simulink model "ARDroneWPTracking_V2"  (R2017b)
settings: Solver=ode1  StartTime=0.0  StopTime=30  FixedStep=sampleTime  RelTol=1e-3  EnableMultiTasking=on
values from neighbouring files (symbols this model uses):
  sampleTime = 1/200    (= 0.005)    [setupHover.m]
libraries: ARBlocks x4
CloseFcn:
  | rtwprivate ssgencode ModelCloseRequest Good_NL_model
settings Model: SimulationMode=external  ExtModeTrigDuration=100000  Creator=Paul  LastModifiedBy=ritac
settings DataIOCC: LimitDataPoints=on  SaveFormat=Array  SignalLoggingSaveFormat=ModelDataLogs  TimeSaveName=time
settings OptimizationCC: ExpressionDepthLimit=2147483647  InitFltsAndDblsToZero=on
settings DebuggingCC: UnderspecifiedInitializationDetection=Classic  MergeDetectMultiDrivingBlocksExec=none  SolverPrmCheckMsg=warning  FcnCallInpInsideContextMsg=warning  StateNameClashWarn=warning  SFUnexpectedBacktrackingDiag=warning  SFNoUnconditionalDefaultTransitionDiag=warning  SFExecutionAtInitializationDiag=none
settings HardwareCC: ProdBitPerLong=64  ProdHWDeviceType=Intel->x86-64 (Mac OS X)
settings ModelReferenceCC: PropagateSignalLabelsOutOfModel=off
settings RTWCC: SystemTargetFile=sldrt.tlc  TemplateMakefile=sldrt.tmf  Description=Simulink Desktop Real-Time  RTWCompilerOptimization=on
settings CodeAppCC: MaxIdLength=95  StateflowObjectComments=on
settings SimulinkDesktopRealTimeCC: TargetPreCompLibLocation=/Applications/MATLAB_R2017b.app/toolbox/sldrt/lib/maci64  TargetLangStandard=C89/C90 (ANSI)  SupportVariableSizeSignals=off
settings ConfigComp: CovMetricSettings=dw  CovHtmlReporting=on  CovSaveCumulativeToWorkspaceVar=on  CovSaveSingleToWorkspaceVar=on  CovExternalEMLEnable=off

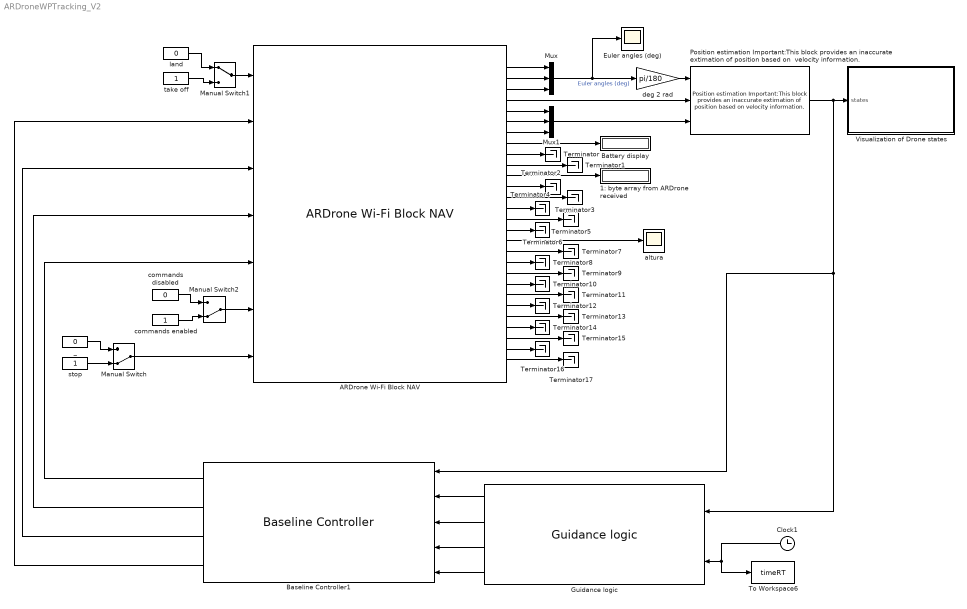
== system ARDroneWPTracking_V2 ==
  "1: byte array from ARDrone received " : Display
  ARDrone Wi-Fi Block NAV : ARBlocks/ARDrone Wi-Fi Block NAV
  Baseline Controller1 : ARBlocks/Baseline Controller
  Battery display : Display
  Clock1 : Clock
  Euler angles (deg) : Scope
  Guidance logic : ARBlocks/Guidance logic
  Manual Switch : ManualSwitch  CurrentSetting=0
  Manual Switch1 : ManualSwitch
  Manual Switch2 : ManualSwitch  CurrentSetting=0
  Mux : Mux  Inputs=3
  Mux1 : Mux  Inputs=3
  "Position estimation Important:This block provides an inaccurate extimation of position based on  velocity information. " : ARBlocks/Position estimation Important:This block provides an  inaccurate extimation of position  based on  velocity information. 
  Terminator{,1..17} (18 alike) : Terminator
  To Workspace6 : ToWorkspace  VariableName=timeRT  SampleTime=sampleTime
  Visualization of Drone states : Subsystem
  _ : Constant  Value=0
  altura : Scope
  commands disabled : Constant  Value=0
  commands enabled : Constant
  deg 2 rad : Gain  Gain=pi/180
  land : Constant  Value=0
  stop : Constant
  take off : Constant
  wires:
  _/1 -> Manual Switch/1
  stop/1 -> Manual Switch/2
  land/1 -> Manual Switch1/1
  take off/1 -> Manual Switch1/2
  commands disabled/1 -> Manual Switch2/1
  commands enabled/1 -> Manual Switch2/2
  Manual Switch1/1 -> ARDrone Wi-Fi Block NAV/1
  Manual Switch2/1 -> ARDrone Wi-Fi Block NAV/6
  Manual Switch/1 -> ARDrone Wi-Fi Block NAV/7
  Baseline Controller1/1 -> ARDrone Wi-Fi Block NAV/5
  Baseline Controller1/3 -> ARDrone Wi-Fi Block NAV/3
  "Position estimation Important:This block provides an inaccurate extimation of position based on  velocity information. "/1 -> Visualization of Drone states/1(states), Guidance logic/1, Baseline Controller1/1
  Clock1/1 -> To Workspace6/1, Guidance logic/2
  Baseline Controller1/4 -> ARDrone Wi-Fi Block NAV/2
  Guidance logic/2 -> Baseline Controller1/3
  Guidance logic/4 -> Baseline Controller1/5
  Guidance logic/1 -> Baseline Controller1/2
  Guidance logic/3 -> Baseline Controller1/4
  Baseline Controller1/2 -> ARDrone Wi-Fi Block NAV/4
  ARDrone Wi-Fi Block NAV/2 -> Mux/2
  ARDrone Wi-Fi Block NAV/18 -> Terminator7/1
  ARDrone Wi-Fi Block NAV/16 -> Terminator6/1
  ARDrone Wi-Fi Block NAV/23 -> Terminator12/1
  ARDrone Wi-Fi Block NAV/28 -> Terminator17/1
  ARDrone Wi-Fi Block NAV/25 -> Terminator14/1
  ARDrone Wi-Fi Block NAV/19 -> Terminator8/1
  ARDrone Wi-Fi Block NAV/26 -> Terminator15/1
  ARDrone Wi-Fi Block NAV/20 -> Terminator9/1
  ARDrone Wi-Fi Block NAV/22 -> Terminator11/1
  ARDrone Wi-Fi Block NAV/12 -> Terminator2/1
  ARDrone Wi-Fi Block NAV/17 -> altura/1
  ARDrone Wi-Fi Block NAV/15 -> Terminator5/1
  Mux1/1 -> "Position estimation Important:This block provides an inaccurate extimation of position based on  velocity information. "/3
  ARDrone Wi-Fi Block NAV/24 -> Terminator13/1
  ARDrone Wi-Fi Block NAV/11 -> "1: byte array from ARDrone received "/1
  ARDrone Wi-Fi Block NAV/1 -> Mux/1
  deg 2 rad/1 -> "Position estimation Important:This block provides an inaccurate extimation of position based on  velocity information. "/1
  ARDrone Wi-Fi Block NAV/21 -> Terminator10/1
  ARDrone Wi-Fi Block NAV/7 -> Mux1/3
  ARDrone Wi-Fi Block NAV/14 -> Terminator4/1
  Mux/1 -> deg 2 rad/1, Euler angles (deg)/1  "Euler angles (deg)"
  ARDrone Wi-Fi Block NAV/4 -> "Position estimation Important:This block provides an inaccurate extimation of position based on  velocity information. "/2
  ARDrone Wi-Fi Block NAV/5 -> Mux1/1
  ARDrone Wi-Fi Block NAV/13 -> Terminator3/1
  ARDrone Wi-Fi Block NAV/9 -> Terminator/1
  ARDrone Wi-Fi Block NAV/27 -> Terminator16/1
  ARDrone Wi-Fi Block NAV/6 -> Mux1/2
  ARDrone Wi-Fi Block NAV/3 -> Mux/3
  ARDrone Wi-Fi Block NAV/10 -> Terminator1/1
  ARDrone Wi-Fi Block NAV/8 -> Battery display/1

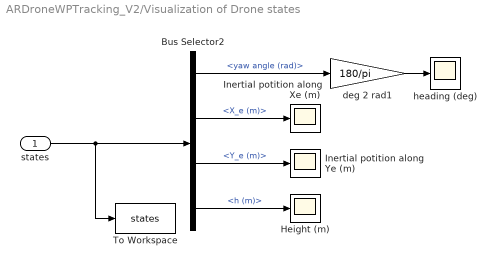
== system ARDroneWPTracking_V2/Visualization of Drone states ==
  states : Inport
  Bus Selector2 : BusSelector  OutputSignals=yaw angle (rad),X_e (m),Y_e (m),h (m)
  Height (m) : Scope
  Inertial potition along Xe (m) : Scope
  Inertial potition along Ye (m) : Scope
  To Workspace : ToWorkspace  VariableName=states  SaveFormat=Structure With Time  SampleTime=-1
  deg 2 rad1 : Gain  Gain=180/pi
  heading (deg) : Scope
  wires:
  states/1 -> To Workspace/1, Bus Selector2/1
  Bus Selector2/1 -> deg 2 rad1/1  "<yaw angle (rad)>"
  Bus Selector2/2 -> Inertial potition along Xe (m)/1  "<X_e (m)>"
  Bus Selector2/3 -> Inertial potition along Ye (m)/1  "<Y_e (m)>"
  Bus Selector2/4 -> Height (m)/1  "<h (m)>"
  deg 2 rad1/1 -> heading (deg)/1
